simulink model "kp_ki_pid"  (R2023a)
settings: Solver=VariableStepAuto  StartTime=0.0  StopTime=10.0  RelTol=1e-3
settings Model: Creator=TUBA  LastModifiedBy=TUBA

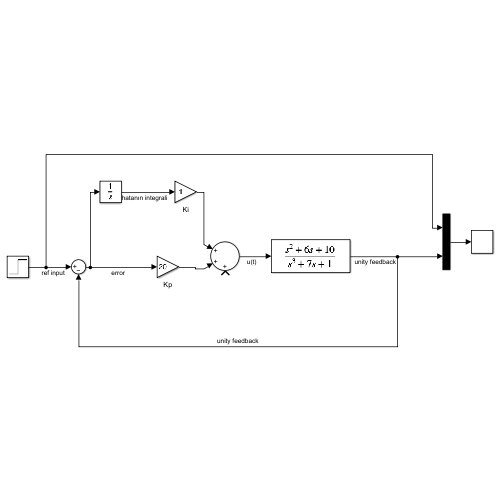
[thumbnail: Simulink's stored preview of the top-level diagram]
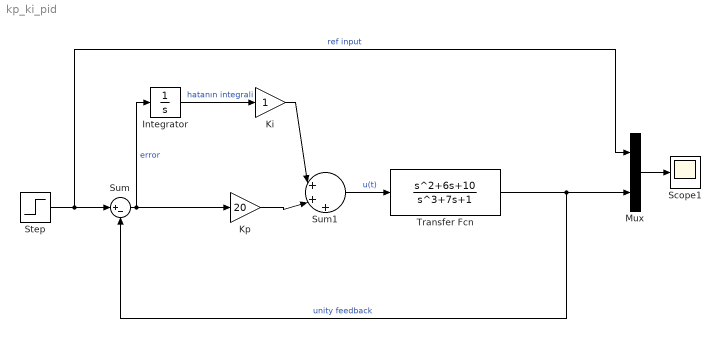
== system kp_ki_pid ==
  Integrator : Integrator
  Ki : Gain
  Kp : Gain  Gain=20
  Mux : Mux  Inputs=2
  Scope1 : Scope
  Step : Step  SampleTime=0
  Sum : Sum  Inputs=|+-
  Sum1 : Sum  Inputs=|+++
  Transfer Fcn : TransferFcn  Numerator=[1,6,10]  Denominator=[1,0,7,1]
  wires:
  Kp/1 -> Sum1/2
  Step/1 -> Mux/1, Sum/1  "ref input"
  Mux/1 -> Scope1/1
  Sum/1 -> Kp/1, Integrator/1  "error"
  Transfer Fcn/1 -> Sum/2, Mux/2  "unity feedback"
  Integrator/1 -> Ki/1  "hatanın integrali"
  Ki/1 -> Sum1/1
  Sum1/1 -> Transfer Fcn/1  "u(t)"
